simulink model "turb_ident1"  (Simulink 4.00)
settings: Solver=ode45  StartTime=0.0  StopTime=100  RelTol=1e-3
settings Model: LastModifiedBy=Administrator  LimitDataPoints=off  BlockReductionOpt=off

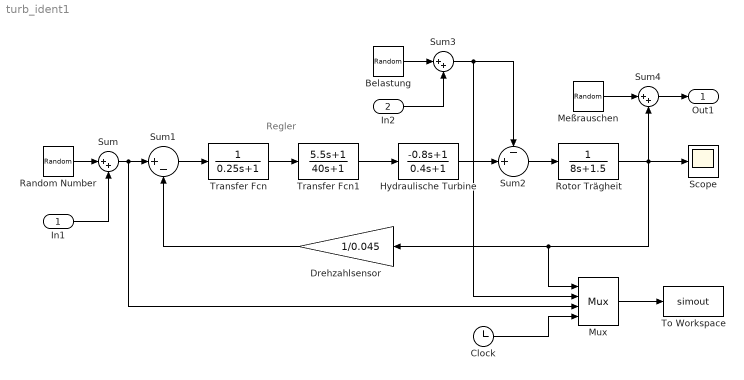
== system turb_ident1 ==
  note: Regler
  In1 : Inport  Port=1
  In2 : Inport  Port=2
  Belastung : RandomNumber  Mean=0  Variance=1  Seed=0  SampleTime=0
  Clock : Clock
      settings: DisplayTime=off  Decimation=10
  Drehzahlsensor : Gain  Orientation=left  Gain=1/0.045  Multiplication=Element-wise(K.*u)  SaturateOnIntegerOverflow=on
  Hydraulische Turbine : TransferFcn  Numerator=[-0.8 1]  Denominator=[0.4 1]  Realization=auto  AbsoluteTolerance=auto
  Meßrauschen : RandomNumber  Mean=0  Variance=1  Seed=0  SampleTime=0
  Mux : Mux  Inputs=4
      settings: DisplayOption=none
  Random Number : RandomNumber  Mean=0  Variance=1  Seed=0  SampleTime=0
  Rotor Trägheit : TransferFcn  Numerator=[1]  Denominator=[8 1.5]  Realization=auto  AbsoluteTolerance=auto
  Scope : Scope
      settings: TimeRange=auto  YMin=-5  YMax=5  SaveToWorkspace=off  SaveName=ScopeData  LimitDataPoints=on  MaxDataPoints=5000
  Sum : Sum  Inputs=|++  SaturateOnIntegerOverflow=on
  Sum1 : Sum  Inputs=|+-  SaturateOnIntegerOverflow=on
  Sum2 : Sum  Inputs=-+|  SaturateOnIntegerOverflow=on
  Sum3 : Sum  Inputs=|++  SaturateOnIntegerOverflow=on
  Sum4 : Sum  Inputs=|++  SaturateOnIntegerOverflow=on
  To Workspace : ToWorkspace  VariableName=simout  SampleTime=-1  SaveFormat=Array
  Transfer Fcn : TransferFcn  Numerator=[1]  Denominator=[0.25 1]  Realization=auto  AbsoluteTolerance=auto
  Transfer Fcn1 : TransferFcn  Numerator=[5.5 1]  Denominator=[40 1]  Realization=auto  AbsoluteTolerance=auto
  Out1 : Outport  Port=1
  wires:
  In1/1 -> Sum/2
  Random Number/1 -> Sum/1
  Sum/1 -> Sum1/1, Mux/3
  Sum1/1 -> Transfer Fcn/1
  Transfer Fcn/1 -> Transfer Fcn1/1
  Transfer Fcn1/1 -> Hydraulische Turbine/1
  Hydraulische Turbine/1 -> Sum2/2
  In2/1 -> Sum3/2
  Belastung/1 -> Sum3/1
  Sum3/1 -> Sum2/1, Mux/2
  Sum2/1 -> Rotor Trägheit/1
  Drehzahlsensor/1 -> Sum1/2
  Rotor Trägheit/1 -> Drehzahlsensor/1, Mux/1, Sum4/2, Scope/1
  Sum4/1 -> Out1/1
  Meßrauschen/1 -> Sum4/1
  Mux/1 -> To Workspace/1
  Clock/1 -> Mux/4
